simulink library "Communication"  (Simulink 7.4)
settings: Solver=ode45  StartTime=0.0  StopTime=10.0  RelTol=1e-3
PostLoadFcn:
  | load CommunicationBus.mat
(part 1 of 2)
settings Model: Creator=dread  LastModifiedBy=dread

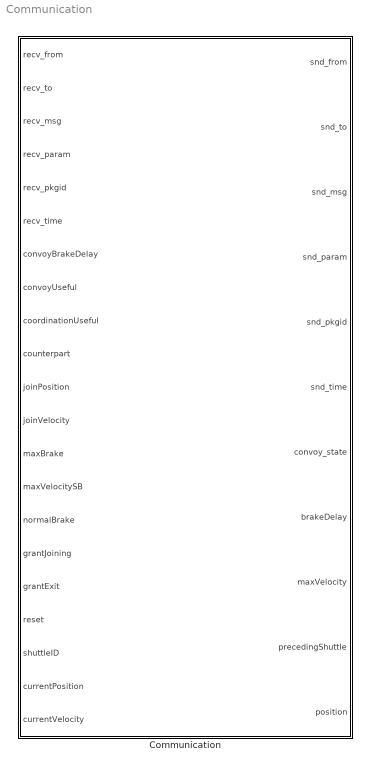
== system Communication ==
  Communication : Subsystem

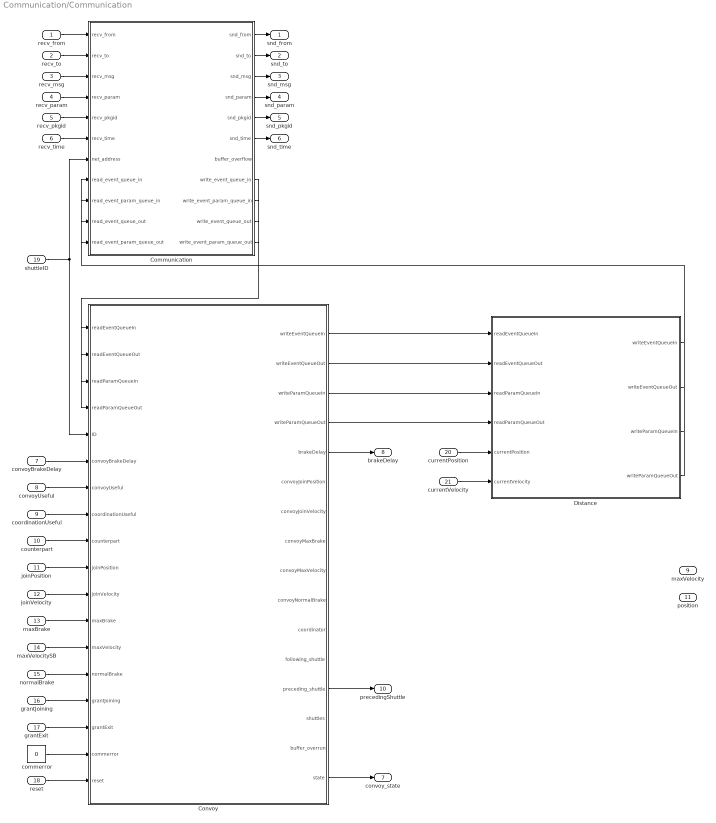
== system Communication/Communication ==
  recv_from : Inport  DataType=uint8  OutDataType=fixdt(1, 16)  OutScaling=2^0  OutDataTypeStr=uint8
  recv_to : Inport  Port=2  DataType=uint8  OutDataType=fixdt(1, 16)  OutScaling=2^0  OutDataTypeStr=uint8
  recv_msg : Inport  Port=3  DataType=uint16  OutDataType=fixdt(1, 16)  OutScaling=2^0  OutDataTypeStr=uint16
  recv_param : Inport  Port=4  DataType=double  OutDataType=fixdt(1, 16)  OutScaling=2^0  OutDataTypeStr=double
  recv_pkgid : Inport  Port=5  DataType=uint32  OutDataType=fixdt(1, 16)  OutScaling=2^0  OutDataTypeStr=uint32
  recv_time : Inport  Port=6  DataType=double  OutDataType=fixdt(1, 16)  OutScaling=2^0  OutDataTypeStr=double
  convoyBrakeDelay : Inport  Port=7  DataType=double  OutDataType=fixdt(1, 16)  OutScaling=2^0  OutDataTypeStr=double
  convoyUseful : Inport  Port=8  DataType=boolean  OutDataType=fixdt(1, 16)  OutScaling=2^0  OutDataTypeStr=boolean
  coordinationUseful : Inport  Port=9  DataType=boolean  OutDataType=fixdt(1, 16)  OutScaling=2^0  OutDataTypeStr=boolean
  counterpart : Inport  Port=10  DataType=double  OutDataType=fixdt(1, 16)  OutScaling=2^0  OutDataTypeStr=double
  joinPosition : Inport  Port=11  DataType=double  OutDataType=fixdt(1, 16)  OutScaling=2^0  OutDataTypeStr=double
  joinVelocity : Inport  Port=12  DataType=double  OutDataType=fixdt(1, 16)  OutScaling=2^0  OutDataTypeStr=double
  maxBrake : Inport  Port=13  DataType=double  OutDataType=fixdt(1, 16)  OutScaling=2^0  OutDataTypeStr=double
  maxVelocitySB : Inport  Port=14  DataType=double  OutDataType=fixdt(1, 16)  OutScaling=2^0  OutDataTypeStr=double
  normalBrake : Inport  Port=15  DataType=double  OutDataType=fixdt(1, 16)  OutScaling=2^0  OutDataTypeStr=double
  grantJoining : Inport  Port=16  OutDataType=fixdt(1, 16)  OutScaling=2^0
  grantExit : Inport  Port=17  OutDataType=fixdt(1, 16)  OutScaling=2^0
  reset : Inport  Port=18  DataType=boolean  OutDataType=fixdt(1, 16)  OutScaling=2^0  OutDataTypeStr=boolean
  shuttleID : Inport  Port=19  OutDataType=fixdt(1, 16)  OutScaling=2^0
  currentPosition : Inport  Port=20  OutDataType=fixdt(1, 16)  OutScaling=2^0
  currentVelocity : Inport  Port=21  OutDataType=fixdt(1, 16)  OutScaling=2^0
  Communication : Subsystem
  Convoy : Subsystem
  Distance : Subsystem
  commerror : Constant  Value=0  OutDataTypeMode=boolean  OutDataType=sfix(16)  OutScaling=2^0  OutDataTypeStr=boolean
  snd_from : Outport  DataType=uint8  OutDataType=fixdt(1, 16)  OutScaling=2^0  OutDataTypeStr=uint8
  snd_to : Outport  Port=2  DataType=uint8  OutDataType=fixdt(1, 16)  OutScaling=2^0  OutDataTypeStr=uint8
  snd_msg : Outport  Port=3  DataType=uint16  OutDataType=fixdt(1, 16)  OutScaling=2^0  OutDataTypeStr=uint16
  snd_param : Outport  Port=4  DataType=double  OutDataType=fixdt(1, 16)  OutScaling=2^0  OutDataTypeStr=double
  snd_pkgid : Outport  Port=5  DataType=uint32  OutDataType=fixdt(1, 16)  OutScaling=2^0  OutDataTypeStr=uint32
  snd_time : Outport  Port=6  DataType=double  OutDataType=fixdt(1, 16)  OutScaling=2^0  OutDataTypeStr=double
  convoy_state : Outport  Port=7  OutDataType=fixdt(1, 16)  OutScaling=2^0
  brakeDelay : Outport  Port=8  OutDataType=fixdt(1, 16)  OutScaling=2^0
  maxVelocity : Outport  Port=9  OutDataType=fixdt(1, 16)  OutScaling=2^0
  precedingShuttle : Outport  Port=10  OutDataType=fixdt(1, 16)  OutScaling=2^0
  position : Outport  Port=11  OutDataType=fixdt(1, 16)  OutScaling=2^0
  wires:
  Distance/3(writeParamQueueIn) -> Communication/9(read_event_param_queue_in)
  Convoy/4(writeParamQueueOut) -> Distance/4(readParamQueueOut)
  Convoy/3(writeParamQueueIn) -> Distance/3(readParamQueueIn)
  Convoy/2(writeEventQueueOut) -> Distance/2(readEventQueueOut)
  Convoy/1(writeEventQueueIn) -> Distance/1(readEventQueueIn)
  Distance/4(writeParamQueueOut) -> Communication/11(read_event_param_queue_out)
  Distance/2(writeEventQueueOut) -> Communication/10(read_event_queue_out)
  Distance/1(writeEventQueueIn) -> Communication/8(read_event_queue_in)
  currentPosition/1 -> Distance/5(currentPosition)
  currentVelocity/1 -> Distance/6(currentVelocity)
  Convoy/13(preceding_shuttle) -> precedingShuttle/1
  Convoy/5(brakeDelay) -> brakeDelay/1
  Convoy/16(state) -> convoy_state/1
  reset/1 -> Convoy/18(reset)
  grantExit/1 -> Convoy/16(grantExit)
  grantJoining/1 -> Convoy/15(grantJoining)
  normalBrake/1 -> Convoy/14(normalBrake)
  maxVelocitySB/1 -> Convoy/13(maxVelocity)
  maxBrake/1 -> Convoy/12(maxBrake)
  joinVelocity/1 -> Convoy/11(joinVelocity)
  joinPosition/1 -> Convoy/10(joinPosition)
  counterpart/1 -> Convoy/9(counterpart)
  coordinationUseful/1 -> Convoy/8(coordinationUseful)
  convoyUseful/1 -> Convoy/7(convoyUseful)
  convoyBrakeDelay/1 -> Convoy/6(convoyBrakeDelay)
  Communication/6(snd_time) -> snd_time/1
  recv_time/1 -> Communication/6(recv_time)
  commerror/1 -> Convoy/17(commerror)
  shuttleID/1 -> Communication/7(net_address), Convoy/5(ID)
  Communication/9(write_event_param_queue_in) -> Convoy/3(readParamQueueIn)
  Communication/11(write_event_param_queue_out) -> Convoy/4(readParamQueueOut)
  Communication/10(write_event_queue_out) -> Convoy/2(readEventQueueOut)
  Communication/8(write_event_queue_in) -> Convoy/1(readEventQueueIn)
  Communication/5(snd_pkgid) -> snd_pkgid/1
  Communication/4(snd_param) -> snd_param/1
  Communication/3(snd_msg) -> snd_msg/1
  Communication/2(snd_to) -> snd_to/1
  Communication/1(snd_from) -> snd_from/1
  recv_pkgid/1 -> Communication/5(recv_pkgid)
  recv_param/1 -> Communication/4(recv_param)
  recv_msg/1 -> Communication/3(recv_msg)
  recv_to/1 -> Communication/2(recv_to)
  recv_from/1 -> Communication/1(recv_from)

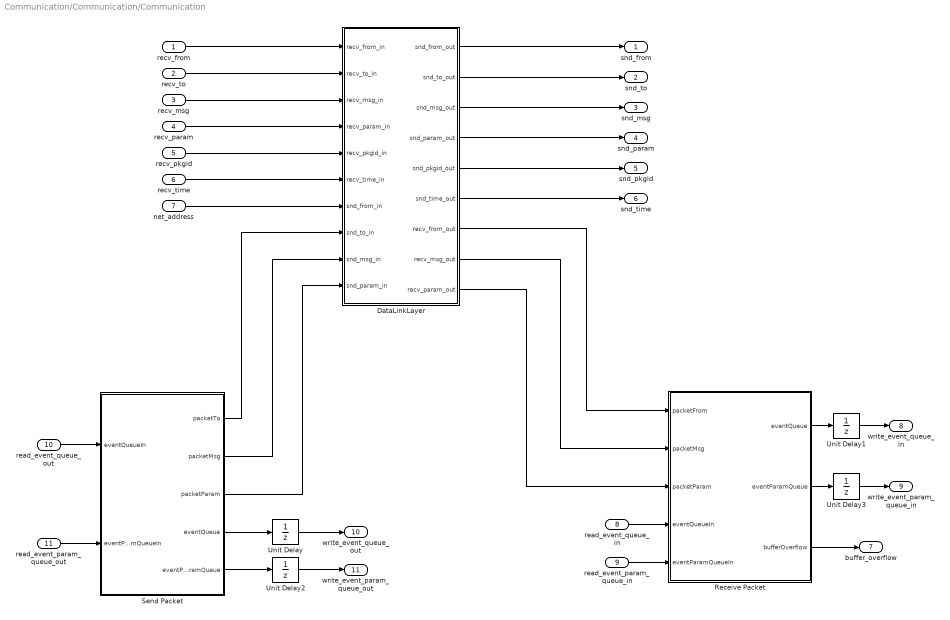
== system Communication/Communication/Communication ==
  recv_from : Inport  DataType=uint8  OutDataType=fixdt(1, 16)  OutScaling=2^0  OutDataTypeStr=uint8
  recv_to : Inport  Port=2  DataType=uint8  OutDataType=fixdt(1, 16)  OutScaling=2^0  OutDataTypeStr=uint8
  recv_msg : Inport  Port=3  DataType=uint16  OutDataType=fixdt(1, 16)  OutScaling=2^0  OutDataTypeStr=uint16
  recv_param : Inport  Port=4  DataType=double  OutDataType=fixdt(1, 16)  OutScaling=2^0  OutDataTypeStr=double
  recv_pkgid : Inport  Port=5  DataType=uint32  OutDataType=fixdt(1, 16)  OutScaling=2^0  OutDataTypeStr=uint32
  recv_time : Inport  Port=6  DataType=double  OutDataType=fixdt(1, 16)  OutScaling=2^0  OutDataTypeStr=double
  net_address : Inport  Port=7  DataType=uint8  OutDataType=fixdt(1, 16)  OutScaling=2^0  OutDataTypeStr=uint8
  read_event_queue_in : Inport  Port=8  PortDimensions=[10,2]  DataType=uint8  OutDataType=fixdt(1, 16)  OutScaling=2^0  OutDataTypeStr=uint8
  read_event_param_queue_in : Inport  Port=9  PortDimensions=[10]  DataType=double  OutDataType=fixdt(1, 16)  OutScaling=2^0  OutDataTypeStr=double
  read_event_queue_out : Inport  Port=10  PortDimensions=[10,2]  DataType=uint8  OutDataType=fixdt(1, 16)  OutScaling=2^0  OutDataTypeStr=uint8
  read_event_param_queue_out : Inport  Port=11  PortDimensions=[10]  DataType=double  OutDataType=fixdt(1, 16)  OutScaling=2^0  OutDataTypeStr=double
  DataLinkLayer : Subsystem
  Receive Packet : Stateflow chart
  Send Packet : Stateflow chart
  Unit Delay{,1..3} (4 alike) : UnitDelay  SampleTime=-1
  snd_from : Outport  DataType=uint8  OutDataType=fixdt(1, 16)  OutScaling=2^0  OutDataTypeStr=uint8
  snd_to : Outport  Port=2  DataType=uint8  OutDataType=fixdt(1, 16)  OutScaling=2^0  OutDataTypeStr=uint8
  snd_msg : Outport  Port=3  DataType=uint16  OutDataType=fixdt(1, 16)  OutScaling=2^0  OutDataTypeStr=uint16
  snd_param : Outport  Port=4  DataType=double  OutDataType=fixdt(1, 16)  OutScaling=2^0  OutDataTypeStr=double
  snd_pkgid : Outport  Port=5  DataType=uint32  OutDataType=fixdt(1, 16)  OutScaling=2^0  OutDataTypeStr=uint32
  snd_time : Outport  Port=6  DataType=double  OutDataType=fixdt(1, 16)  OutScaling=2^0  OutDataTypeStr=double
  buffer_overflow : Outport  Port=7  DataType=boolean  OutDataType=fixdt(1, 16)  OutScaling=2^0  OutDataTypeStr=boolean
  write_event_queue_in : Outport  Port=8  PortDimensions=[10,2]  DataType=uint8  OutDataType=fixdt(1, 16)  OutScaling=2^0  OutDataTypeStr=uint8
  write_event_param_queue_in : Outport  Port=9  PortDimensions=[10]  DataType=double  OutDataType=fixdt(1, 16)  OutScaling=2^0  OutDataTypeStr=double
  write_event_queue_out : Outport  Port=10  PortDimensions=[10,2]  DataType=uint8  OutDataType=fixdt(1, 16)  OutScaling=2^0  OutDataTypeStr=uint8
  write_event_param_queue_out : Outport  Port=11  PortDimensions=[10]  DataType=double  OutDataType=fixdt(1, 16)  OutScaling=2^0  OutDataTypeStr=double
  wires:
  Unit Delay3/1 -> write_event_param_queue_in/1
  Unit Delay1/1 -> write_event_queue_in/1
  Unit Delay2/1 -> write_event_param_queue_out/1
  Unit Delay/1 -> write_event_queue_out/1
  read_event_queue_out/1 -> Send Packet/1(eventQueueIn)
  read_event_param_queue_out/1 -> Send Packet/2(eventParamQueueIn)
  net_address/1 -> DataLinkLayer/7(snd_from_in)
  recv_time/1 -> DataLinkLayer/6(recv_time_in)
  recv_pkgid/1 -> DataLinkLayer/5(recv_pkgid_in)
  recv_param/1 -> DataLinkLayer/4(recv_param_in)
  recv_msg/1 -> DataLinkLayer/3(recv_msg_in)
  recv_to/1 -> DataLinkLayer/2(recv_to_in)
  recv_from/1 -> DataLinkLayer/1(recv_from_in)
  DataLinkLayer/6(snd_time_out) -> snd_time/1
  Send Packet/3(packetParam) -> DataLinkLayer/10(snd_param_in)
  Send Packet/2(packetMsg) -> DataLinkLayer/9(snd_msg_in)
  Send Packet/1(packetTo) -> DataLinkLayer/8(snd_to_in)
  Send Packet/5(eventParamQueue) -> Unit Delay2/1
  Send Packet/4(eventQueue) -> Unit Delay/1
  Receive Packet/3(bufferOverflow) -> buffer_overflow/1
  Receive Packet/2(eventParamQueue) -> Unit Delay3/1
  Receive Packet/1(eventQueue) -> Unit Delay1/1
  read_event_param_queue_in/1 -> Receive Packet/5(eventParamQueueIn)
  read_event_queue_in/1 -> Receive Packet/4(eventQueueIn)
  DataLinkLayer/9(recv_param_out) -> Receive Packet/3(packetParam)
  DataLinkLayer/8(recv_msg_out) -> Receive Packet/2(packetMsg)
  DataLinkLayer/7(recv_from_out) -> Receive Packet/1(packetFrom)
  DataLinkLayer/5(snd_pkgid_out) -> snd_pkgid/1
  DataLinkLayer/4(snd_param_out) -> snd_param/1
  DataLinkLayer/3(snd_msg_out) -> snd_msg/1
  DataLinkLayer/2(snd_to_out) -> snd_to/1
  DataLinkLayer/1(snd_from_out) -> snd_from/1

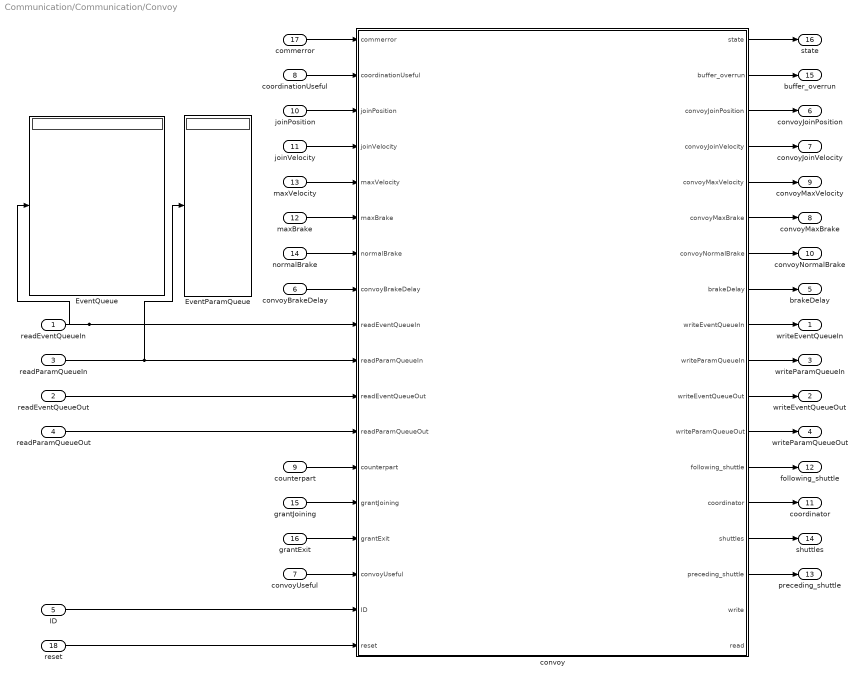
== system Communication/Communication/Convoy ==
  readEventQueueIn : Inport  DataType=uint8  OutDataType=fixdt(1, 16)  OutScaling=2^0  OutDataTypeStr=uint8
  readEventQueueOut : Inport  Port=2  DataType=uint8  OutDataType=fixdt(1, 16)  OutScaling=2^0  OutDataTypeStr=uint8
  readParamQueueIn : Inport  Port=3  DataType=double  OutDataType=fixdt(1, 16)  OutScaling=2^0  OutDataTypeStr=double
  readParamQueueOut : Inport  Port=4  DataType=double  OutDataType=fixdt(1, 16)  OutScaling=2^0  OutDataTypeStr=double
  ID : Inport  Port=5  DataType=uint8  OutDataType=fixdt(1, 16)  OutScaling=2^0  OutDataTypeStr=uint8
  convoyBrakeDelay : Inport  Port=6  DataType=double  OutDataType=fixdt(1, 16)  OutScaling=2^0  OutDataTypeStr=double
  convoyUseful : Inport  Port=7  DataType=boolean  OutDataType=fixdt(1, 16)  OutScaling=2^0  OutDataTypeStr=boolean
  coordinationUseful : Inport  Port=8  DataType=boolean  OutDataType=fixdt(1, 16)  OutScaling=2^0  OutDataTypeStr=boolean
  counterpart : Inport  Port=9  DataType=double  OutDataType=fixdt(1, 16)  OutScaling=2^0  OutDataTypeStr=double
  joinPosition : Inport  Port=10  DataType=double  OutDataType=fixdt(1, 16)  OutScaling=2^0  OutDataTypeStr=double
  joinVelocity : Inport  Port=11  DataType=double  OutDataType=fixdt(1, 16)  OutScaling=2^0  OutDataTypeStr=double
  maxBrake : Inport  Port=12  DataType=double  OutDataType=fixdt(1, 16)  OutScaling=2^0  OutDataTypeStr=double
  maxVelocity : Inport  Port=13  DataType=double  OutDataType=fixdt(1, 16)  OutScaling=2^0  OutDataTypeStr=double
  normalBrake : Inport  Port=14  DataType=double  OutDataType=fixdt(1, 16)  OutScaling=2^0  OutDataTypeStr=double
  grantJoining : Inport  Port=15  OutDataType=fixdt(1, 16)  OutScaling=2^0
  grantExit : Inport  Port=16  OutDataType=fixdt(1, 16)  OutScaling=2^0
  commerror : Inport  Port=17  DataType=boolean  OutDataType=fixdt(1, 16)  OutScaling=2^0  OutDataTypeStr=boolean
  reset : Inport  Port=18  DataType=boolean  OutDataType=fixdt(1, 16)  OutScaling=2^0  OutDataTypeStr=boolean
  EventParamQueue : Display
  EventQueue : Display
  "convoy " : Stateflow chart  TreatAsAtomicUnit=on
  writeEventQueueIn : Outport  DataType=uint8  OutDataType=fixdt(1, 16)  OutScaling=2^0  OutDataTypeStr=uint8
  writeEventQueueOut : Outport  Port=2  DataType=uint8  OutDataType=fixdt(1, 16)  OutScaling=2^0  OutDataTypeStr=uint8
  writeParamQueueIn : Outport  Port=3  DataType=double  OutDataType=fixdt(1, 16)  OutScaling=2^0  OutDataTypeStr=double
  writeParamQueueOut : Outport  Port=4  DataType=double  OutDataType=fixdt(1, 16)  OutScaling=2^0  OutDataTypeStr=double
  brakeDelay : Outport  Port=5  DataType=double  OutDataType=fixdt(1, 16)  OutScaling=2^0  OutDataTypeStr=double
  convoyJoinPosition : Outport  Port=6  DataType=double  OutDataType=fixdt(1, 16)  OutScaling=2^0  OutDataTypeStr=double
  convoyJoinVelocity : Outport  Port=7  DataType=double  OutDataType=fixdt(1, 16)  OutScaling=2^0  OutDataTypeStr=double
  convoyMaxBrake : Outport  Port=8  DataType=double  OutDataType=fixdt(1, 16)  OutScaling=2^0  OutDataTypeStr=double
  convoyMaxVelocity : Outport  Port=9  DataType=double  OutDataType=fixdt(1, 16)  OutScaling=2^0  OutDataTypeStr=double
  convoyNormalBrake : Outport  Port=10  DataType=double  OutDataType=fixdt(1, 16)  OutScaling=2^0  OutDataTypeStr=double
  coordinator : Outport  Port=11  DataType=uint8  OutDataType=fixdt(1, 16)  OutScaling=2^0  OutDataTypeStr=uint8
  following_shuttle : Outport  Port=12  DataType=uint8  OutDataType=fixdt(1, 16)  OutScaling=2^0  OutDataTypeStr=uint8
  preceding_shuttle : Outport  Port=13  DataType=uint8  OutDataType=fixdt(1, 16)  OutScaling=2^0  OutDataTypeStr=uint8
  shuttles : Outport  Port=14  DataType=uint8  OutDataType=fixdt(1, 16)  OutScaling=2^0  OutDataTypeStr=uint8
  buffer_overrun : Outport  Port=15  DataType=boolean  OutDataType=fixdt(1, 16)  OutScaling=2^0  OutDataTypeStr=boolean
  state : Outport  Port=16  DataType=uint8  OutDataType=fixdt(1, 16)  OutScaling=2^0  OutDataTypeStr=uint8
  wires:
  grantExit/1 -> "convoy "/15(grantExit)
  grantJoining/1 -> "convoy "/14(grantJoining)
  convoyBrakeDelay/1 -> "convoy "/8(convoyBrakeDelay)
  "convoy "/16(preceding_shuttle) -> preceding_shuttle/1
  "convoy "/15(shuttles) -> shuttles/1
  "convoy "/14(coordinator) -> coordinator/1
  "convoy "/13(following_shuttle) -> following_shuttle/1
  "convoy "/12(writeParamQueueOut) -> writeParamQueueOut/1
  "convoy "/11(writeEventQueueOut) -> writeEventQueueOut/1
  "convoy "/10(writeParamQueueIn) -> writeParamQueueIn/1
  "convoy "/9(writeEventQueueIn) -> writeEventQueueIn/1
  "convoy "/8(brakeDelay) -> brakeDelay/1
  "convoy "/7(convoyNormalBrake) -> convoyNormalBrake/1
  "convoy "/6(convoyMaxBrake) -> convoyMaxBrake/1
  "convoy "/5(convoyMaxVelocity) -> convoyMaxVelocity/1
  "convoy "/4(convoyJoinVelocity) -> convoyJoinVelocity/1
  "convoy "/3(convoyJoinPosition) -> convoyJoinPosition/1
  "convoy "/2(buffer_overrun) -> buffer_overrun/1
  "convoy "/1(state) -> state/1
  counterpart/1 -> "convoy "/13(counterpart)
  convoyUseful/1 -> "convoy "/16(convoyUseful)
  joinPosition/1 -> "convoy "/3(joinPosition)
  joinVelocity/1 -> "convoy "/4(joinVelocity)
  maxVelocity/1 -> "convoy "/5(maxVelocity)
  maxBrake/1 -> "convoy "/6(maxBrake)
  normalBrake/1 -> "convoy "/7(normalBrake)
  coordinationUseful/1 -> "convoy "/2(coordinationUseful)
  commerror/1 -> "convoy "/1(commerror)
  ID/1 -> "convoy "/17(ID)
  reset/1 -> "convoy "/18(reset)
  readParamQueueOut/1 -> "convoy "/12(readParamQueueOut)
  readParamQueueIn/1 -> "convoy "/10(readParamQueueIn), EventParamQueue/1
  readEventQueueOut/1 -> "convoy "/11(readEventQueueOut)
  readEventQueueIn/1 -> "convoy "/9(readEventQueueIn), EventQueue/1

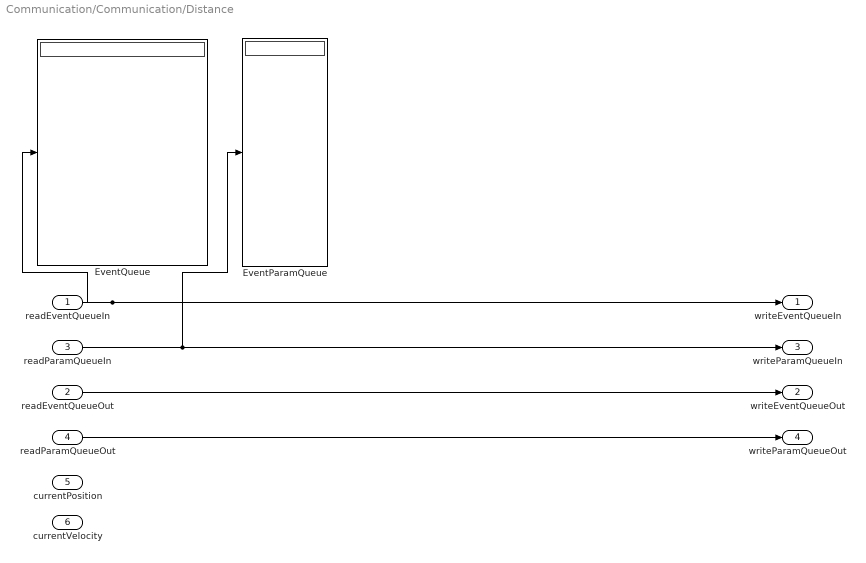
== system Communication/Communication/Distance ==
  readEventQueueIn : Inport  DataType=uint8  OutDataType=fixdt(1, 16)  OutScaling=2^0  OutDataTypeStr=uint8
  readEventQueueOut : Inport  Port=2  DataType=uint8  OutDataType=fixdt(1, 16)  OutScaling=2^0  OutDataTypeStr=uint8
  readParamQueueIn : Inport  Port=3  DataType=double  OutDataType=fixdt(1, 16)  OutScaling=2^0  OutDataTypeStr=double
  readParamQueueOut : Inport  Port=4  DataType=double  OutDataType=fixdt(1, 16)  OutScaling=2^0  OutDataTypeStr=double
  currentPosition : Inport  Port=5  OutDataType=fixdt(1, 16)  OutScaling=2^0
  currentVelocity : Inport  Port=6  OutDataType=fixdt(1, 16)  OutScaling=2^0
  EventParamQueue : Display
  EventQueue : Display
  writeEventQueueIn : Outport  DataType=uint8  OutDataType=fixdt(1, 16)  OutScaling=2^0  OutDataTypeStr=uint8
  writeEventQueueOut : Outport  Port=2  DataType=uint8  OutDataType=fixdt(1, 16)  OutScaling=2^0  OutDataTypeStr=uint8
  writeParamQueueIn : Outport  Port=3  DataType=double  OutDataType=fixdt(1, 16)  OutScaling=2^0  OutDataTypeStr=double
  writeParamQueueOut : Outport  Port=4  DataType=double  OutDataType=fixdt(1, 16)  OutScaling=2^0  OutDataTypeStr=double
  wires:
  readParamQueueOut/1 -> writeParamQueueOut/1
  readParamQueueIn/1 -> writeParamQueueIn/1, EventParamQueue/1
  readEventQueueOut/1 -> writeEventQueueOut/1
  readEventQueueIn/1 -> writeEventQueueIn/1, EventQueue/1

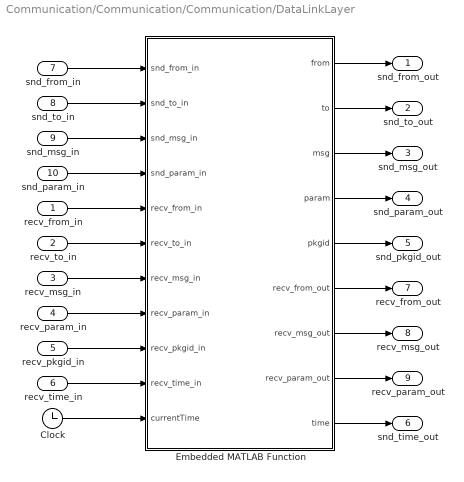
== system Communication/Communication/Communication/DataLinkLayer ==
  recv_from_in : Inport  DataType=uint8  OutDataType=fixdt(1, 16)  OutScaling=2^0  OutDataTypeStr=uint8
  recv_to_in : Inport  Port=2  DataType=uint8  OutDataType=fixdt(1, 16)  OutScaling=2^0  OutDataTypeStr=uint8
  recv_msg_in : Inport  Port=3  DataType=uint16  OutDataType=fixdt(1, 16)  OutScaling=2^0  OutDataTypeStr=uint16
  recv_param_in : Inport  Port=4  DataType=double  OutDataType=fixdt(1, 16)  OutScaling=2^0  OutDataTypeStr=double
  recv_pkgid_in : Inport  Port=5  DataType=uint32  OutDataType=fixdt(1, 16)  OutScaling=2^0  OutDataTypeStr=uint32
  recv_time_in : Inport  Port=6  DataType=double  OutDataType=fixdt(1, 16)  OutScaling=2^0  OutDataTypeStr=double
  snd_from_in : Inport  Port=7  DataType=uint8  OutDataType=fixdt(1, 16)  OutScaling=2^0  OutDataTypeStr=uint8
  snd_to_in : Inport  Port=8  DataType=uint8  OutDataType=fixdt(1, 16)  OutScaling=2^0  OutDataTypeStr=uint8
  snd_msg_in : Inport  Port=9  DataType=uint16  OutDataType=fixdt(1, 16)  OutScaling=2^0  OutDataTypeStr=uint16
  snd_param_in : Inport  Port=10  DataType=double  OutDataType=fixdt(1, 16)  OutScaling=2^0  OutDataTypeStr=double
  Clock : Clock
      settings: Decimation=10
  Embedded MATLAB Function : Stateflow chart
  snd_from_out : Outport  DataType=uint8  OutDataType=fixdt(1, 16)  OutScaling=2^0  OutDataTypeStr=uint8
  snd_to_out : Outport  Port=2  DataType=uint8  OutDataType=fixdt(1, 16)  OutScaling=2^0  OutDataTypeStr=uint8
  snd_msg_out : Outport  Port=3  DataType=uint16  OutDataType=fixdt(1, 16)  OutScaling=2^0  OutDataTypeStr=uint16
  snd_param_out : Outport  Port=4  DataType=double  OutDataType=fixdt(1, 16)  OutScaling=2^0  OutDataTypeStr=double
  snd_pkgid_out : Outport  Port=5  DataType=uint32  OutDataType=fixdt(1, 16)  OutScaling=2^0  OutDataTypeStr=uint32
  snd_time_out : Outport  Port=6  DataType=double  OutDataType=fixdt(1, 16)  OutScaling=2^0  OutDataTypeStr=double
  recv_from_out : Outport  Port=7  DataType=uint8  OutDataType=fixdt(1, 16)  OutScaling=2^0  OutDataTypeStr=uint8
  recv_msg_out : Outport  Port=8  DataType=uint16  OutDataType=fixdt(1, 16)  OutScaling=2^0  OutDataTypeStr=uint16
  recv_param_out : Outport  Port=9  DataType=double  OutDataType=fixdt(1, 16)  OutScaling=2^0  OutDataTypeStr=double
  wires:
  Clock/1 -> Embedded MATLAB Function/11(currentTime)
  Embedded MATLAB Function/9(time) -> snd_time_out/1
  recv_time_in/1 -> Embedded MATLAB Function/10(recv_time_in)
  recv_pkgid_in/1 -> Embedded MATLAB Function/9(recv_pkgid_in)
  recv_param_in/1 -> Embedded MATLAB Function/8(recv_param_in)
  recv_msg_in/1 -> Embedded MATLAB Function/7(recv_msg_in)
  recv_to_in/1 -> Embedded MATLAB Function/6(recv_to_in)
  recv_from_in/1 -> Embedded MATLAB Function/5(recv_from_in)
  Embedded MATLAB Function/8(recv_param_out) -> recv_param_out/1
  Embedded MATLAB Function/7(recv_msg_out) -> recv_msg_out/1
  Embedded MATLAB Function/6(recv_from_out) -> recv_from_out/1
  snd_to_in/1 -> Embedded MATLAB Function/2(snd_to_in)
  snd_from_in/1 -> Embedded MATLAB Function/1(snd_from_in)
  snd_param_in/1 -> Embedded MATLAB Function/4(snd_param_in)
  snd_msg_in/1 -> Embedded MATLAB Function/3(snd_msg_in)
  Embedded MATLAB Function/5(pkgid) -> snd_pkgid_out/1
  Embedded MATLAB Function/4(param) -> snd_param_out/1
  Embedded MATLAB Function/3(msg) -> snd_msg_out/1
  Embedded MATLAB Function/2(to) -> snd_to_out/1
  Embedded MATLAB Function/1(from) -> snd_from_out/1

== matlab function Communication/Communication/Receive Packet ==
  data: packetFrom input double; packetMsg input double; packetParam input double; eventQueueIn input double; eventParamQueueIn input double; eventQueue output double; eventParamQueue output double; bufferOverflow output boolean
function [eventQueue, eventParamQueue, bufferOverflow] = receivePacket(packetFrom, packetMsg, packetParam, eventQueueIn, eventParamQueueIn)
%#eml
% This function receives packets and adds them to the event queue.
% A packet consists of a source, a message and an optional parameter for 
% the message. Source and message are contained at position 1 and 2 in the 
% eventQueue. Because of the different data type the parameter has his own 
% queue eventParamQueue.

%Constants
SOURCE = 2;
MESSAGE = 1;

%Init
eventQueue = eventQueueIn;
eventParamQueue = eventParamQueueIn;
bufferOverflow = false;

%New incoming packet
if packetFrom ~= 0
    %Add it to the incoming event Queue
    for i = 1:length(eventQueue)
        %Search for an empty place
        if eventQueue(i,SOURCE) == 0
            eventQueue(i,SOURCE)    = packetFrom;
            eventQueue(i,MESSAGE)   = packetMsg;
            eventParamQueue(i)      = packetParam;
            return;
        end
    end
    %No empty place found
    bufferOverflow = true;
end

== matlab function Communication/Communication/Send Packet ==
  data: packetTo output double; packetMsg output double; packetParam output double; eventQueue output double; eventParamQueue output double; eventQueueIn input double; eventParamQueueIn input double
function [packetTo, packetMsg, packetParam, eventQueue, eventParamQueue] = sendPacket(eventQueueIn, eventParamQueueIn)
%#eml
eml.extrinsic('disp');
% This function creates packets from the event queue. A packet consists
% of a destination, a message and an optional parameter for the message.
% Destination and message are contained at position 1 and 2 in the 
% eventQueue. Because of the different data type the parameter has his own 
% queue eventParamQueue.

%Constants
DESTINATION = 2;
MESSAGE = 1;

%Init
eventQueue = eventQueueIn;
eventParamQueue = eventParamQueueIn;
packetTo = uint8(0);
packetMsg = uint16(0);
packetParam = 0;

%There is an event in the queue
if eventQueue(1,DESTINATION) ~= 0
    %Create packet from the firs entry in the queue
    packetTo    = eventQueue(1,DESTINATION);
    packetMsg   = uint16(eventQueue(1,MESSAGE));
    packetParam = eventParamQueue(1);
    %Remove the event from the queue
    for i=1:length(eventQueue) - 1
        eventQueue(i,DESTINATION)   = eventQueue(i+1,DESTINATION);
        eventQueue(i,MESSAGE)       = eventQueue(i+1,MESSAGE);
        eventParamQueue(i)          = eventParamQueue(i+1);
    end
    %Set last element to zero
    eventQueue(length(eventQueue),DESTINATION)  = 0;
    eventQueue(length(eventQueue),MESSAGE)      = 0;
    eventParamQueue(length(eventParamQueue))    = 0;
end

== matlab function Communication/Communication/DataLinkLayer/Embedded MATLAB Function ==
  data: snd_from_in input double; snd_to_in input double; snd_msg_in input double; snd_param_in input double; from output double; to output double; msg output double; param output double; pkgid output double; recv_from_in input double; recv_to_in input double; recv_msg_in input double; recv_param_in input double; recv_pkgid_in input double; recv_from_out output double; recv_msg_out output double; recv_param_out output double; recv_time_in input double; time output double; currentTime input double
function [from, to, msg, param, pkgid, recv_from_out, recv_msg_out, recv_param_out, time] = ackHandler(snd_from_in, snd_to_in, snd_msg_in, snd_param_in, recv_from_in, recv_to_in, recv_msg_in, recv_param_in, recv_pkgid_in, recv_time_in, currentTime)
%#eml
eml.extrinsic('warning', 'disp');

%Init
from    = uint8(0);
to      = uint8(0);
msg     = uint16(0);
param   = 0;
pkgid   = uint32(0);
time    = 0;
 
recv_from_out    = uint8(0);
recv_msg_out     = uint16(0);
recv_param_out   = 0;


snd_in = packet(snd_from_in, snd_to_in, snd_msg_in, snd_param_in, 0, 0);
recv_in = packet(recv_from_in, recv_to_in, recv_msg_in, recv_param_in, recv_pkgid_in, recv_time_in);

%Constants
TIMEOUT_ACK     = 2.0;
MSG_ACK         = 255;
QUEUE_SIZE_SENDING = 10;
QUEUE_SIZE_ACK  = 10;
QUEUE_SIZE_RECEIVED = 10;

%Persistent variables
persistent pkgidCounter sendingQueue ackQueue receivedQueue

if isempty(pkgidCounter)
    pkgidCounter = uint32(1);
end

if isempty(sendingQueue)
    sendingQueue = repmat(packet(0,0,0,0,0,0), 1, QUEUE_SIZE_SENDING);
end

if isempty(ackQueue)
    ackQueue = repmat(packet(0,0,0,0,0,0), 1, QUEUE_SIZE_ACK);
end

if isempty(receivedQueue)
    receivedQueue = repmat(packet(0, 0, 0, 0, 0, 0), 1, QUEUE_SIZE_RECEIVED);
end


%Step 1: Check for a new outgoing packet
if snd_in.to ~= 0        
    %Add packet id
    snd_in.pkgid = pkgidCounter;
    %Increment packet counter
    pkgidCounter = pkgidCounter + 1;   
    %Set time
    snd_in.time = currentTime;
    %Add packet so the outgoing queue
    sendingQueue = enqueue(sendingQueue, snd_in);      
end

%Step 2: Check for a new incoming packet
if recv_in.from ~= 0
    if recv_in.msg == MSG_ACK
        %Remove packet from ackQueue
        for i=1:length(ackQueue)
            if ackQueue(i).pkgid == uint8(recv_in.param)
                ackQueue = dequeue(ackQueue,i);
                break;
            end
        end
    else
        %Send ACK
        ackPacket = packet(recv_in.to, recv_in.from, MSG_ACK, double(recv_in.pkgid),pkgidCounter, currentTime);
        pkgidCounter = pkgidCounter + 1;
        sendingQueue = enqueue(sendingQueue,ackPacket);
        
        %Check for duplicated packets
        duplicatedPacket = false;
        for i=1:length(receivedQueue)
            if receivedQueue(i).pkgid == recv_in.pkgid && receivedQueue(i).from == recv_in.from
                duplicatedPacket = true;
                break;
            end
        end
        
        if duplicatedPacket == false
            %forward packet
            recv_from_out    = recv_in.from;
            recv_msg_out     = recv_in.msg;
            recv_param_out   = recv_in.param;
            
            %check if received queue is full, remove packet
            if receivedQueue(length(receivedQueue)).from ~= 0
                receivedQueue = dequeue(receivedQueue,1);
            end
            
            %save packet            
            receivedQueue = enqueue(receivedQueue, recv_in);
            
        end
    end
end


%Step 3: Timeout reached? Send packet again
for i = 1:length(ackQueue)
    if ackQueue(i).to ~= 0
        if ackQueue(i).time + TIMEOUT_ACK <= currentTime
            %Reset counter
            ackQueue(i).time = currentTime;
            %Send again
            sendingQueue = enqueue(sendingQueue, ackQueue(i));
            %Remove packet from ackQueue
            ackQueue = dequeue(ackQueue, i);
        end
    end
end


%Step 4: Send outgoing packet
if sendingQueue(1).to ~= 0    
    from    = sendingQueue(1).from;
    to      = sendingQueue(1).to;
    msg     = sendingQueue(1).msg;
    param   = sendingQueue(1).param;
    pkgid   = sendingQueue(1).pkgid;
    time    = sendingQueue(1).time;
    
    %Add it to the ack queue
    if sendingQueue(1).msg ~= MSG_ACK
        ackQueue = enqueue(ackQueue, sendingQueue(1));
    end
    
    %remove packet from sending queue
    sendingQueue = dequeue(sendingQueue, 1);    
end


%%%%%%%%%%%%%%%%%%%%%%%%%%%%%%%%%%%%%%%%%%%%%%%%%%%%%%%%%%%%%%%%%%%%%%%%%%%
%%                          H E L P E R
%%%%%%%%%%%%%%%%%%%%%%%%%%%%%%%%%%%%%%%%%%%%%%%%%%%%%%%%%%%%%%%%%%%%%%%%%%%

function p = packet(from, to, msg, param, pkgid, time)
%#eml
%Defines a packet
p = struct('from', uint8(from),'to', uint8(to),'msg', uint16(msg),'param', double(param),'pkgid', uint32(pkgid), 'time', double(time));


function queue = enqueue(queue, packet)
%#eml
eml.extrinsic('warning');
for i = 1:length(queue)
    if queue(i).to == 0
        queue(i) = packet;
        return;
    end
end
warning('RailCab:DataLinkLayer', 'Buffer overflow');

function queue = dequeue(queue, index)
%#eml
assert(index <= length(queue))
for i=index:length(queue)-1;
    queue(i) = queue(i+1);
end
queue(length(queue)) = packet(0,0,0,0,0,0);
